simulink model "twsbr_lqr"  (R2026a)
settings: Solver=ode45  StopTime=8.0  MaxStep=0.001  RelTol=1e-9  AbsTol=1e-11
model workspace (MAT data in the model file):
  disturbance_force_data = [0  0; 8  0]
  disturbance_torque_data = [0  0; 8  0]
  position_reference_data = [0  0; 8  0]
settings Model: Creator=Linxiuqi  LastModifiedBy=Linxiuqi

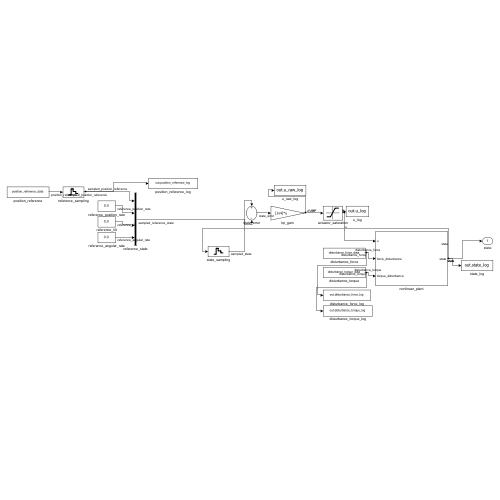
[thumbnail: Simulink's stored preview of the top-level diagram]
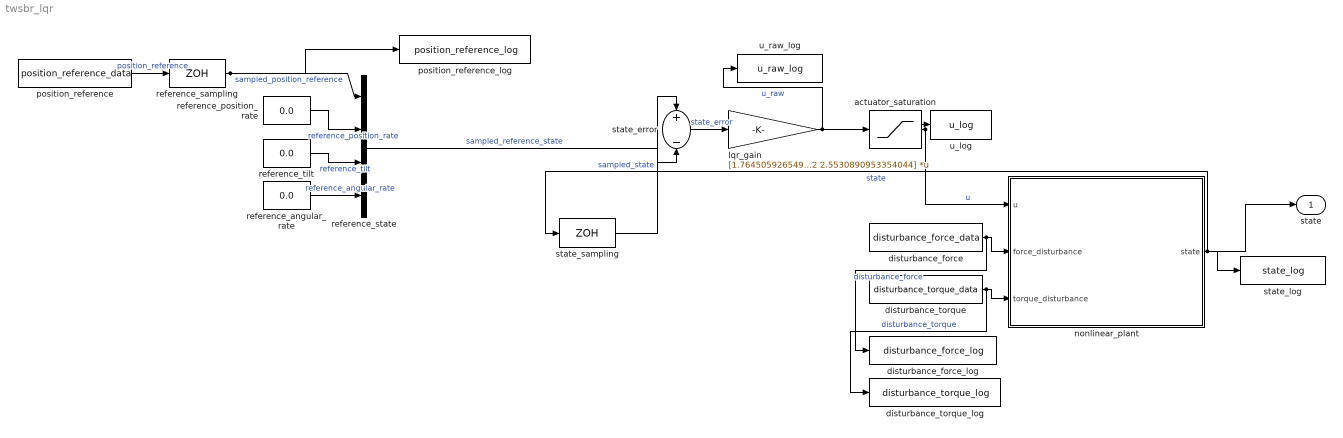
== system twsbr_lqr ==
  actuator_saturation : Saturate  UpperLimit=1  LowerLimit=-1
  disturbance_force : FromWorkspace  VariableName=disturbance_force_data  Interpolate=off  OutputAfterFinalValue=Holding final value
  disturbance_force_log : ToWorkspace  VariableName=disturbance_force_log  SaveFormat=Structure With Time  SampleTime=-1
  disturbance_torque : FromWorkspace  VariableName=disturbance_torque_data  Interpolate=off  OutputAfterFinalValue=Holding final value
  disturbance_torque_log : ToWorkspace  VariableName=disturbance_torque_log  SaveFormat=Structure With Time  SampleTime=-1
  lqr_gain : Gain  Gain=[1.7645059265494396 2.2042597811313396 13.816371986143462 2.5530890953354044]  Multiplication=Matrix(K*u)
  nonlinear_plant : Subsystem
  position_reference : FromWorkspace  VariableName=position_reference_data  Interpolate=off  OutputAfterFinalValue=Holding final value
  position_reference_log : ToWorkspace  VariableName=position_reference_log  SaveFormat=Structure With Time  SampleTime=-1
  reference_angular_rate : Constant  Value=0.0
  reference_position_rate : Constant  Value=0.0
  reference_sampling : ZeroOrderHold  SampleTime=0.01
  reference_state : Mux
  reference_tilt : Constant  Value=0.0
  state_error : Sum  Inputs=+-
  state_log : ToWorkspace  VariableName=state_log  SaveFormat=Structure With Time  SampleTime=-1
  state_sampling : ZeroOrderHold  SampleTime=0.01
  u_log : ToWorkspace  VariableName=u_log  SaveFormat=Structure With Time  SampleTime=-1
  u_raw_log : ToWorkspace  VariableName=u_raw_log  SaveFormat=Structure With Time  SampleTime=-1
  state : Outport
  wires:
  position_reference/1 -> reference_sampling/1  "position_reference"
  reference_sampling/1 -> reference_state/1, position_reference_log/1  "sampled_position_reference"
  reference_position_rate/1 -> reference_state/2  "reference_position_rate"
  reference_tilt/1 -> reference_state/3  "reference_tilt"
  reference_angular_rate/1 -> reference_state/4  "reference_angular_rate"
  reference_state/1 -> state_error/2  "sampled_reference_state"
  nonlinear_plant/1(state) -> state_sampling/1, state/1, state_log/1  "state"
  state_sampling/1 -> state_error/1  "sampled_state"
  state_error/1 -> lqr_gain/1  "state_error"
  lqr_gain/1 -> actuator_saturation/1, u_raw_log/1  "u_raw"
  actuator_saturation/1 -> nonlinear_plant/1(u), u_log/1  "u"
  disturbance_force/1 -> nonlinear_plant/2(force_disturbance), disturbance_force_log/1  "disturbance_force"
  disturbance_torque/1 -> nonlinear_plant/3(torque_disturbance), disturbance_torque_log/1  "disturbance_torque"

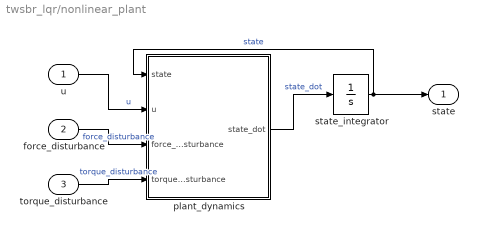
== system twsbr_lqr/nonlinear_plant ==
  u : Inport
  force_disturbance : Inport  Port=2
  torque_disturbance : Inport  Port=3
  plant_dynamics : MATLAB Function  TreatAsAtomicUnit=on
  state_integrator : Integrator  InitialCondition=[0;0;0;0]
  state : Outport
  wires:
  plant_dynamics/1(state_dot) -> state_integrator/1  "state_dot"
  torque_disturbance/1 -> plant_dynamics/4(torque_disturbance)  "torque_disturbance"
  force_disturbance/1 -> plant_dynamics/3(force_disturbance)  "force_disturbance"
  u/1 -> plant_dynamics/2(u)  "u"
  state_integrator/1 -> state/1, plant_dynamics/1(state)  "state"

== matlab function twsbr_lqr/nonlinear_plant/plant_dynamics ==
  data: state input; u input; state_dot output; force_disturbance input; torque_disturbance input
function state_dot = plant_dynamics(state, u, force_disturbance, torque_disturbance)
%#codegen
body_mass = 1.2;
wheel_mass = 0.29999999999999999;
com_length = 0.17999999999999999;
body_inertia = 0.025000000000000001;
damping = 0.050000000000000003;
gravity = 9.8100000000000005;
motor_gain = 12;
x_dot = state(2);
theta = state(3);
theta_dot = state(4);
force = motor_gain * u + force_disturbance;
mass_sum = wheel_mass + body_mass;
rotational_term = body_inertia + body_mass * com_length^2;
coupling = body_mass * com_length * cos(theta);
rhs_position = force - damping * x_dot + body_mass * com_length * theta_dot^2 * sin(theta);
rhs_angle = body_mass * gravity * com_length * sin(theta) + torque_disturbance;
determinant = mass_sum * rotational_term - coupling^2;
x_ddot = (rotational_term * rhs_position - coupling * rhs_angle) / determinant;
theta_ddot = (-coupling * rhs_position + mass_sum * rhs_angle) / determinant;
state_dot = [x_dot; x_ddot; theta_dot; theta_ddot];
end
